simulink model "OSQP"  (R2025a)
settings: Solver=ode8  StartTime=0.0  StopTime=1  FixedStep=100e-6  RelTol=1e-3
settings Model: Creator=JR  LastModifiedBy=JR

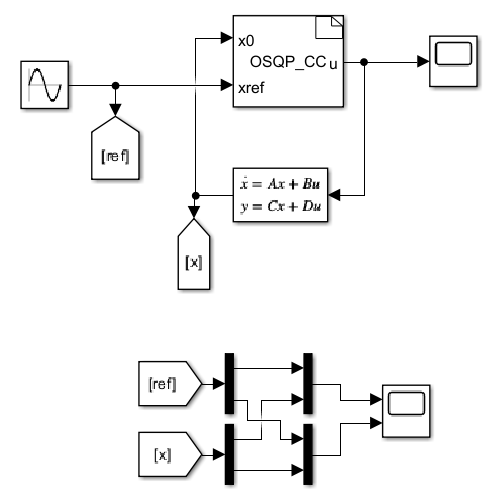
[thumbnail: Simulink's stored preview of the top-level diagram]
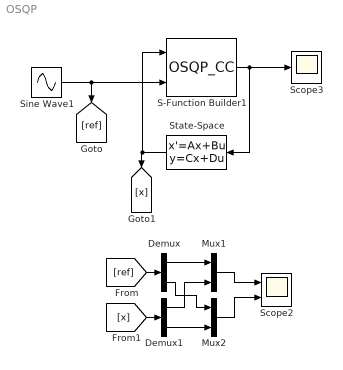
== system OSQP ==
  Demux : Demux  Outputs=2
  Demux1 : Demux  Outputs=2
  Mux1 : Mux  Inputs=2
  Mux2 : Mux  Inputs=2
  S-Function Builder1 : S-Function  FunctionName=OSQP_CC  SFunctionModules=OSQP_CC_wrapper.c cpg_workspace cpg_solve workspace emosqp algebra_libs auxil csc_math csc_utils error kkt matrix osqp_api qdldl qdldl_interface scaling util vector  SFunctionDeploymentMode=off  EnableBusSupport=off  mask(S-Function Builder){}
      mask help: Simulink:masks:SFunctionBuilder_MD
      mask init:
      | val = [[.9  0.75 0.75 1 1 .9 .9 1]',[1 1 0.75 0.75 .9 .9 1 .9]'];try , sys = get_param(gcb,'SfunBuilderFcnName');if isempty(sys), sys = get_param(gcb,'FunctionName'); end,catch, sys = get_param(gcb,'FunctionName'); end
      settings: CopyFcn=set_param(gcbh,'LinkStatus','none')  OpenFcn=sfunctionwizard(gcbh)
      mask Display:
      | plot(val(:,1),val(:,2))
      | disp(sys)
      | port_label('input',1,sprintf('%s', 'x0'),'interpreter','tex')
      | port_label('input',2,sprintf('%s', 'xref'),'interpreter','tex')
      | port_label('output',1,sprintf('%s', 'u'),'interpreter','tex')
  Scope2 : Scope  NumInputPorts=2
      settings: ActiveDisplayYMinimum=-2.4999999680253175  ActiveDisplayYMaximum=2.4999999964472575  DataLoggingVariableName=ScopeData2
  Scope3 : Scope
      settings: ActiveDisplayYMinimum=-38.46153851475038  ActiveDisplayYMaximum=38.46153851475038  DataLoggingVariableName=ScopeData3
  Sine Wave1 : Sin  Amplitude=[1;1]  Frequency=100  Phase=[0;pi/2]  SampleTime=0
  State-Space : StateSpace  A=[0 0;0 0]  B=[-400 0; 0 -400]  C=[1 0;0 1]  D=[0 0;0 0]  InitialCondition=[2 ;-1]
  wires:
  [ref] -> Demux/1
  Sine Wave1/1 -> S-Function Builder1/2, [ref]
  Mux2/1 -> Scope2/2
  State-Space/1 -> S-Function Builder1/1, [x]
  Mux1/1 -> Scope2/1
  S-Function Builder1/1 -> State-Space/1, Scope3/1
  Demux1/2 -> Mux2/2
  Demux1/1 -> Mux1/2
  [x] -> Demux1/1
  Demux/2 -> Mux2/1
  Demux/1 -> Mux1/1
